simulink model "TestMultirotorSimPx4v1_8"  (R2018b)
settings: Solver=VariableStepAuto  StartTime=0.0  StopTime=Simulation.T_END  MaxStep=Simulation.TS_MAX  RelTol=1e-3  EnableMultiTasking=on
PreLoadFcn:
  | % InitializeParameters;
undefined symbols (not defined in the file): Aero, armed, ctrl_state, Initial, Motor, Simulation, Uav, v_att_sp, v_control_mode
libraries: QuaternionLibrary x13, simulink_extras x9, Px4Library x3, dspsigattribs x1, dspstat3 x1, simulink x1
(part 2 of 9)

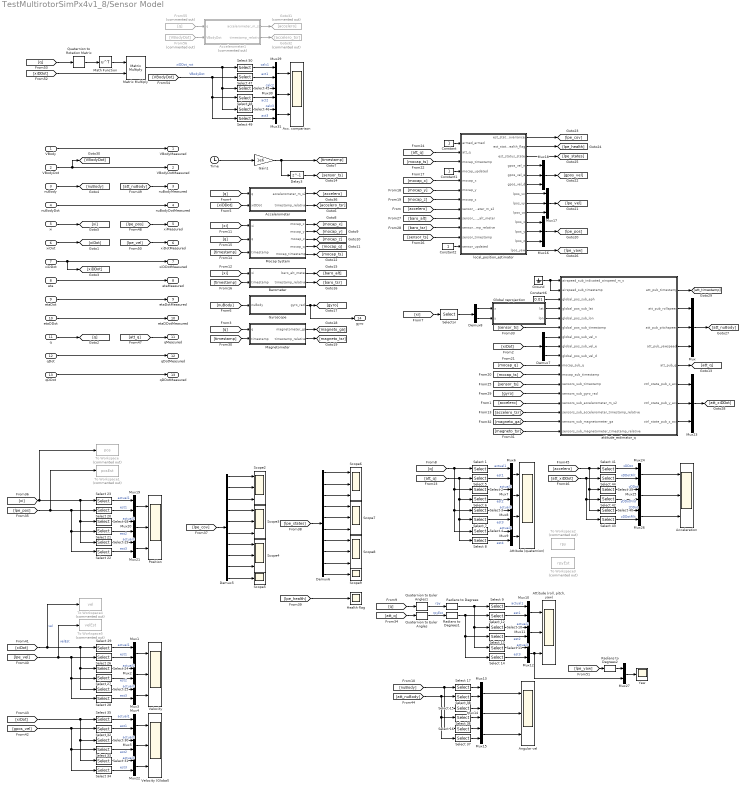
== system TestMultirotorSimPx4v1_8/Sensor Model ==
  VBody : Inport  Unit=m/s  PortDimensions=3
  VBodyDot : Inport  Port=2  Unit=m/s^2  PortDimensions=3
  nuBody : Inport  Port=3  Unit=rad/s  PortDimensions=3
  nuBodyDot : Inport  Port=4  Unit=rad/s^2  PortDimensions=3
  xi : Inport  Port=5  Unit=m  PortDimensions=3
  xiDot : Inport  Port=6  Unit=m/s  PortDimensions=3
  xiDDot : Inport  Port=7  Unit=m/s^2  PortDimensions=3
  eta : Inport  Port=8  Unit=rad  PortDimensions=3
  etaDot : Inport  Port=9  Unit=rad/s  PortDimensions=3
  etaDDot : Inport  Port=10  Unit=rad/s^2  PortDimensions=3
  q : Inport  Port=11  PortDimensions=4
  qDot : Inport  Port=12  PortDimensions=4
  qDDot : Inport  Port=13  PortDimensions=4
  Acc. comparison : Scope  NumInputPorts=3
  Acceleration : Scope  NumInputPorts=3
  Accelerometer : Subsystem
  Accelerometer1 : Subsystem  Commented=on
  Angular vel : Scope  NumInputPorts=3
  Attitude (quaternion) : Scope  NumInputPorts=4
  "Attitude (roll, pitch, yaw)" : Scope  NumInputPorts=3
  Barometer : Subsystem
  Constant : Constant
  Constant1 : Constant
  Constant2 : Constant
  Constant6 : Constant  Value=0.01
  Delay3 : Delay  DelayLength=1  SampleTime=1/400
  Demux5 : Demux  Outputs=10
  Demux6 : Demux  Outputs=10
  Demux7 : Demux  Outputs=3
  Demux8 : Demux  Outputs=2
  From55 : From  Commented=on  GotoTag=q
  From56 : From  Commented=on  GotoTag=VBodyDot
  Gain1 : Gain  Gain=1e6
  Global reprojection : Subsystem  AncestorBlock=Px4Library/Global reprojection  mask{LAT0=-36.865577, LON0=174.772065}
      mask prompts: LAT0 "Latitude at [x,y] = [0,0]"; LON0 "Longitude at [x,y] = [0,0]"
      mask Display:
      | disp('REPROJECT')
      | port_label('input', 1, sprintf('x'))
      | port_label('input', 2, sprintf('y'))
      | port_label('output', 1, sprintf('lat'))
      | port_label('output', 2, sprintf('lon'))
  Goto31 : Goto  Commented=on  GotoTag=accelero
  Goto32 : Goto  Commented=on  GotoTag=accelero_tsr
  Ground : Ground
  Gyroscope : Subsystem
  Health flag : Scope
  Magnetometer : Subsystem
  Math Function : Math  Operator=transpose  SaturateOnIntegerOverflow=on
  Matrix Multiply : Product  Multiplication=Matrix(*)
  Mocap System : Subsystem
  Mux{,16..18,23} (5 alike) : Mux  Inputs=3
  Mux{1..15,19..22,24..27,29..31} (26 alike) : Mux  Inputs=2
  Position : Scope  NumInputPorts=3
  Quaternion to Euler Angles : QuaternionLibrary/Quaternion to Euler Angles
  Quaternion to Euler Angles1 : QuaternionLibrary/Quaternion to Euler Angles
  Quaternion to Rotation Matrix : QuaternionLibrary/Quaternion to Rotation Matrix
  Radians to Degrees : simulink_extras/Transformations/Radians to Degrees
  Radians to Degrees1 : simulink_extras/Transformations/Radians to Degrees
  Radians to Degrees2 : simulink_extras/Transformations/Radians to Degrees
  Scope{2..4,6..8} (6 alike) : Scope  NumInputPorts=3
  Scope5 : Scope
  Scope9 : Scope
  Select 1 : Selector  InputPortWidth=4  IndexOptions=Index vector (dialog)  Indices=1  OutputSizes=1
  Select {10,13,15,18,21,24,27,30,33,36,39,42,45,48} (14 alike) : Selector  InputPortWidth=3  IndexOptions=Index vector (dialog)  Indices=2  OutputSizes=1
  Select {11,14,16,19,22,25,28,31,34,37,40,43,46,49} (14 alike) : Selector  InputPortWidth=3  IndexOptions=Index vector (dialog)  Indices=3  OutputSizes=1
  Select {9,12,17,20,23,26,29,32,35,38,41,44,47,50} (14 alike) : Selector  InputPortWidth=3  IndexOptions=Index vector (dialog)  Indices=1  OutputSizes=1
  Select 2 : Selector  InputPortWidth=4  IndexOptions=Index vector (dialog)  Indices=2  OutputSizes=1
  Select 3 : Selector  InputPortWidth=4  IndexOptions=Index vector (dialog)  Indices=3  OutputSizes=1
  Select 4 : Selector  InputPortWidth=4  IndexOptions=Index vector (dialog)  Indices=4  OutputSizes=1
  Select 5 : Selector  InputPortWidth=4  IndexOptions=Index vector (dialog)  Indices=1  OutputSizes=1
  Select 6 : Selector  InputPortWidth=4  IndexOptions=Index vector (dialog)  Indices=2  OutputSizes=1
  Select 7 : Selector  InputPortWidth=4  IndexOptions=Index vector (dialog)  Indices=3  OutputSizes=1
  Select 8 : Selector  InputPortWidth=4  IndexOptions=Index vector (dialog)  Indices=4  OutputSizes=1
  Selector : Selector  InputPortWidth=3  IndexOptions=Index vector (dialog)  Indices=[1 2]  OutputSizes=1
  Time : Clock
  To Workspace : ToWorkspace  Commented=on  VariableName=pos  SaveFormat=Structure With Time  SampleTime=-1
  To Workspace1 : ToWorkspace  Commented=on  VariableName=posEst  SaveFormat=Structure With Time  SampleTime=-1
  To Workspace2 : ToWorkspace  Commented=on  VariableName=rpy  SaveFormat=Structure With Time  SampleTime=-1
  To Workspace3 : ToWorkspace  Commented=on  VariableName=rpyEst  SaveFormat=Structure With Time  SampleTime=-1
  To Workspace4 : ToWorkspace  Commented=on  VariableName=vel  SaveFormat=Structure With Time  SampleTime=-1
  To Workspace5 : ToWorkspace  Commented=on  VariableName=velEst  SaveFormat=Structure With Time  SampleTime=-1
  Velocity : Scope  NumInputPorts=3
  Velocity (Global) : Scope  NumInputPorts=3
  Yaw : Scope
  attitude_estimator_q : Subsystem  AncestorBlock=Px4Library/attitude_estimator_q  mask(PX4 LPE (local position estimator): local_position_estimator){Q_SAMPLING_PERIOD=1/250, INIT_Q=[1  0  0  0], ATT_W_ACC=0.2, ATT_W_MAG=0.1, ATT_W_EXT_HDG=0.1, ATT_W_GYRO_BIAS=0.1, ATT_MAG_DECL=0.0, ATT_MAG_DECL_A=1, ATT_EXT_HDG_M=2, ATT_ACC_COMP=1, ATT_BIAS_MAX=0.05, FW_ARSP_MODE=0}
      mask prompts: Q_SAMPLING_PERIOD "Sampling period (s)"; INIT_Q "INIT_Q - Initial UAV orientation - set to 0 to let controller decide (bugged) (-)"; ATT_W_ACC "ATT_W_ACC - Complimentary filter accelerometer weight (-)"; ATT_W_MAG "ATT_W_MAG - Complimentary filter magnetometer weight (-)"; ATT_W_EXT_HDG "ATT_W_EXT_HDG - Complimentary filter external heading weight (-)"; ATT_W_GYRO_BIAS "ATT_W_GYRO_BIAS - Complimentary filter gyroscope bias weight (-)"; ATT_MAG_DECL "ATT_MAG_DECL - Magnetic declination. Not used when GPS available (deg)"; ATT_MAG_DECL_A "ATT_MAG_DECL_A - Automatic GPS based declination compensation (-)"; ATT_EXT_HDG_M "ATT_EXT_HDG_M - External heading usage mode (from Motion capture/Vision) (-), 0 None 1 Vision 2 Motion Capture"; ATT_ACC_COMP "ATT_ACC_COMP - Acceleration compensation based on GPS velocity. (-)"; ATT_BIAS_MAX "ATT_BIAS_MAX - Gyro bias limit (rad/s)"; FW_ARSP_MODE "FW_ARSP_MODE - Method used to publish the airspeed (-), 0 Measured airspeed 1 Vehicle ground speed 2 Airspeed invalid"
      mask TypeOptions ATT_EXT_HDG_M: 0 | 1 | 2
      mask TypeOptions FW_ARSP_MODE: 0 | 1 | 2
  local_position_estimator : Subsystem  AncestorBlock=Px4Library/local_position_estimator  mask(PX4 LPE (local position estimator): local_position_estimator){LPE_SAMPLING_PERIOD=0.01, LPE_ACC_XY=0.012, LPE_ACC_Z=0.02, LPE_BAR_Z=3, LPE_EPH_MAX=3, LPE_EPV_MAX=5, LPE_FAKE_ORIGIN=0, LPE_FGYRO_HP=0.001, LPE_FLW_OFF_Z=0, LPE_FLW_QMIN=150, LPE_FLW_R=7, LPE_FLW_RR=7, LPE_FLW_SCALE=1.3, LPE_GPS_DELAY=0.29, LPE_GPS_VXY=0.25, LPE_GPS_VZ=0.25, LPE_GPS_XY=1, LPE_GPS_Z=3, LPE_LAND_VXY=0.05, LPE_LAND_Z=0.03, LPE_LAT=47.3977, LPE_LDR_OFF_Z=0, LPE_LDR_Z=0.03, LPE_LON=8.5456, LPE_PN_B=0.001, LPE_PN_P=0.1, LPE_PN_T=0.001, LPE_PN_V=0.1, LPE_SNR_OFF_Z=0, LPE_SNR_Z=0.05, LPE_T_MAX_GRADE=1, LPE_VIC_P=0.001, LPE_VIS_DELAY=0.1, LPE_VIS_XY=0.1, LPE_VIS_Z=0.5, LPE_VXY_PUB=0.3, LPE_X_LP=5, LPE_Z_PUB=1, LPE_FUSION=193, Barometer=on, GPS=off, LIDAR=off, Flow=off, Sonar=off, Vision=off, Mocap=on, Land=on}
      mask prompts: LPE_SAMPLING_PERIOD "Sampling period (s)"; LPE_ACC_XY "LPE_ACC_XY - Accelerometer xy noise density (m/s^2/sqrt(Hz))"; LPE_ACC_Z "LPE_ACC_Z - Accelerometer z noise density (m/s^2/sqrt(Hz))"; LPE_BAR_Z "LPE_BAR_Z - Barometric presssure altitude z standard deviation. (m)"; LPE_EPH_MAX "LPE_EPH_MAX - Max EPH allowed for GPS initialization (m)"; LPE_EPV_MAX "LPE_EPV_MAX - Max EPV allowed for GPS initialization (m)"; LPE_FAKE_ORIGIN "LPE_FAKE_ORIGIN - Enable publishing of a fake global position (e.g for AUTO missions using Optical Flow) (-)"; LPE_FGYRO_HP "LPE_FGYRO_HP - Flow gyro high pass filter cut off frequency (Hz)"; LPE_FLW_OFF_Z "LPE_FLW_OFF_Z - Optical flow z offset from center (m)"; LPE_FLW_QMIN "LPE_FLW_QMIN - Optical flow minimum quality threshold (-)"; LPE_FLW_R "LPE_FLW_R - Optical flow rotation (roll/pitch) noise gain (m/s / (rad))"; LPE_FLW_RR "LPE_FLW_RR - Optical flow angular velocity noise gain (m/s / (rad/s))"; LPE_FLW_SCALE "LPE_FLW_SCALE - Optical flow scale (m)"; LPE_GPS_DELAY "LPE_GPS_DELAY - GPS delay compensaton (sec)"; LPE_GPS_VXY "LPE_GPS_VXY - GPS xy velocity standard deviation. (m/s)"; LPE_GPS_VZ "LPE_GPS_VZ - GPS z velocity standard deviation. (m/s)"; LPE_GPS_XY "LPE_GPS_XY - Minimum GPS xy standard deviation, uses reported EPH if greater. (m)"; LPE_GPS_Z "LPE_GPS_Z - Minimum GPS z standard deviation, uses reported EPV if greater. (m)"; LPE_LAND_VXY "LPE_LAND_VXY - Land detector xy velocity standard deviation (m/s)"; LPE_LAND_Z "LPE_LAND_Z - Land detector z standard deviation (m)"; LPE_LAT "LPE_LAT - Local origin latitude for nav w/o GPS (deg)"; LPE_LDR_OFF_Z "LPE_LDR_OFF_Z - Lidar z offset from center of vehicle +down (m)"; LPE_LDR_Z "LPE_LDR_Z - Lidar z standard deviation. (m)"; LPE_LON "LPE_LON - Local origin longitude for nav w/o GPS (deg)"; LPE_PN_B "LPE_PN_B - Accel bias propagation noise density ((m/s^2)/s/sqrt(Hz))"; LPE_PN_P "LPE_PN_P - Position propagation noise density (m/s/sqrt(Hz))"; LPE_PN_T "LPE_PN_T - Terrain random walk noise density, hilly/outdoor (0.1), flat/Indoor (0.001) ((m/s)/(sqrt(hz)))"; LPE_PN_V "LPE_PN_V - Velocity propagation noise density ((m/s)/s/sqrt(Hz))"; LPE_SNR_OFF_Z "LPE_SNR_OFF_Z - Sonar z offset from center of vehicle +down (m)"; LPE_SNR_Z "LPE_SNR_Z - Sonar z standard deviation. (m)"; LPE_T_MAX_GRADE "LPE_T_MAX_GRADE - Terrain maximum percent grade, hilly/outdoor (100 = 45 deg), flat/Indoor (0 = 0 deg) (%)"; LPE_VIC_P "LPE_VIC_P - Vicon position standard deviation. (m)"; LPE_VIS_DELAY "LPE_VIS_DELAY - Vision delay compensaton. (sec)"; LPE_VIS_XY "LPE_VIS_XY - Vision xy standard deviation. (m)"; LPE_VIS_Z "LPE_VIS_Z - Vision z standard deviation. (m)"; LPE_VXY_PUB "LPE_VXY_PUB - Required velocity xy standard deviation to publish position (m/s)"; LPE_X_LP "LPE_X_LP - Cut frequency for state publication (Hz)"; LPE_Z_PUB "LPE_Z_PUB - Required z standard deviation to publish altitude/ terrain (m)"; LPE_FUSION "LPE_FUSION - Integer bitmask controlling data fusion (-)"; Barometer "Use Barometer"; GPS "Use GPS"; LIDAR "Use LIDAR"; Flow "Use Flow"; Sonar "Use Sonar"; Vision "Use Vision"; Mocap "Use Mocap"; Land "Use Land"
      mask Callback Barometer:
      | status = get_param( gcb, 'Barometer' );
      | if strcmp( status, 'on' )
      | 	lpe = bitor( uint8(str2num(get_param( gcb, 'LPE_FUSION' ))), uint8(2^0) );
      | 	set_param( gcb, 'LPE_FUSION', num2str(lpe) );
      | else
      | 	lpe = bitand( uint8(str2num(get_param( gcb, 'LPE_FUSION' ))), bitcmp(uint8(2^0), 'uint8' ));
      | 	set_param( gcb, 'LPE_FUSION', num2str(lpe) );
      | end
      mask Callback GPS:
      | status = get_param( gcb, 'GPS' );
      | if strcmp( status, 'on' )
      | 	lpe = bitor( uint8(str2num(get_param( gcb, 'LPE_FUSION' ))), uint8(2^1) );
      | 	set_param( gcb, 'LPE_FUSION', num2str(lpe) );
      | else
      | 	lpe = bitand( uint8(str2num(get_param( gcb, 'LPE_FUSION' ))), bitcmp(uint8(2^1), 'uint8' ));
      | 	set_param( gcb, 'LPE_FUSION', num2str(lpe) );
      | end
      mask Callback LIDAR:
      | status = get_param( gcb, 'LIDAR' );
      | if strcmp( status, 'on' )
      | 	lpe = bitor( uint8(str2num(get_param( gcb, 'LPE_FUSION' ))), uint8(2^2) );
      | 	set_param( gcb, 'LPE_FUSION', num2str(lpe) );
      | else
      | 	lpe = bitand( uint8(str2num(get_param( gcb, 'LPE_FUSION' ))), bitcmp(uint8(2^2), 'uint8' ));
      | 	set_param( gcb, 'LPE_FUSION', num2str(lpe) );
      | end
      mask Callback Flow:
      | status = get_param( gcb, 'Flow' );
      | if strcmp( status, 'on' )
      | 	lpe = bitor( uint8(str2num(get_param( gcb, 'LPE_FUSION' ))), uint8(2^3) );
      | 	set_param( gcb, 'LPE_FUSION', num2str(lpe) );
      | else
      | 	lpe = bitand( uint8(str2num(get_param( gcb, 'LPE_FUSION' ))), bitcmp(uint8(2^3), 'uint8' ));
      | 	set_param( gcb, 'LPE_FUSION', num2str(lpe) );
      | end
      mask Callback Sonar:
      | status = get_param( gcb, 'Sonar' );
      | if strcmp( status, 'on' )
      | 	lpe = bitor( uint8(str2num(get_param( gcb, 'LPE_FUSION' ))), uint8(2^4) );
      | 	set_param( gcb, 'LPE_FUSION', num2str(lpe) );
      | else
      | 	lpe = bitand( uint8(str2num(get_param( gcb, 'LPE_FUSION' ))), bitcmp(uint8(2^4), 'uint8' ));
      | 	set_param( gcb, 'LPE_FUSION', num2str(lpe) );
      | end
      mask Callback Vision:
      | status = get_param( gcb, 'Vision' );
      | if strcmp( status, 'on' )
      | 	lpe = bitor( uint8(str2num(get_param( gcb, 'LPE_FUSION' ))), uint8(2^5) );
      | 	set_param( gcb, 'LPE_FUSION', num2str(lpe) );
      | else
      | 	lpe = bitand( uint8(str2num(get_param( gcb, 'LPE_FUSION' ))), bitcmp(uint8(2^5), 'uint8' ));
      | 	set_param( gcb, 'LPE_FUSION', num2str(lpe) );
      | end
      mask Callback Mocap:
      | status = get_param( gcb, 'Mocap' );
      | if strcmp( status, 'on' )
      | 	lpe = bitor( uint8(str2num(get_param( gcb, 'LPE_FUSION' ))), uint8(2^6) );
      | 	set_param( gcb, 'LPE_FUSION', num2str(lpe) );
      | else
      | 	lpe = bitand( uint8(str2num(get_param( gcb, 'LPE_FUSION' ))), bitcmp(uint8(2^6), 'uint8' ));
      | 	set_param( gcb, 'LPE_FUSION', num2str(lpe) );
      | end
      mask Callback Land:
      | status = get_param( gcb, 'Land' );
      | if strcmp( status, 'on' )
      | 	lpe = bitor( uint8(str2num(get_param( gcb, 'LPE_FUSION' ))), uint8(2^7) );
      | 	set_param( gcb, 'LPE_FUSION', num2str(lpe) );
      | else
      | 	lpe = bitand( uint8(str2num(get_param( gcb, 'LPE_FUSION' ))), bitcmp(uint8(2^7), 'uint8' ));
      | 	set_param( gcb, 'LPE_FUSION', num2str(lpe) );
      | end
  VBodyMeasured : Outport  Unit=m/s
  VBodyDotMeasured : Outport  Port=2  Unit=m/s^2
  nuBodyMeasured : Outport  Port=3  Unit=rad/s
  nuBodyDotMeasured : Outport  Port=4  Unit=rad/s^2
  xiMeasured : Outport  Port=5  Unit=m
  xiDotMeasured : Outport  Port=6  Unit=m/s
  xiDDotMeasured : Outport  Port=7  Unit=m/s^2
  etaMeasured : Outport  Port=8  Unit=rad
  etaDotMeasured : Outport  Port=9  Unit=rad/s
  etaDDotMeasured : Outport  Port=10  Unit=rad/s^2
  qMeasured : Outport  Port=11
  qDotMeasured : Outport  Port=12
  qDDotMeasured : Outport  Port=13
  gyro : Outport  Port=14
  wires:
  xiDot/1 -> [xiDot]
  xi/1 -> [xi]
  nuBodyDot/1 -> nuBodyDotMeasured/1
  nuBody/1 -> [nuBody]
  VBodyDot/1 -> [VBodyDot], VBodyDotMeasured/1
  VBody/1 -> VBodyMeasured/1
  eta/1 -> etaMeasured/1
  etaDot/1 -> etaDotMeasured/1
  etaDDot/1 -> etaDDotMeasured/1
  q/1 -> [q]
  qDot/1 -> qDotMeasured/1
  qDDot/1 -> qDDotMeasured/1
  [att_q] -> local_position_estimator/2(att_q)
  [mocap_x] -> local_position_estimator/5(mocap_x)
  [mocap_z] -> local_position_estimator/7(mocap_z)
  local_position_estimator/10(lpos_x) -> Mux16/1
  local_position_estimator/11(lpos_y) -> Mux16/2
  local_position_estimator/12(lpos_z) -> Mux16/3
  Demux5/2 -> Scope2/2
  Demux5/1 -> Scope2/1
  Demux5/3 -> Scope2/3
  Demux5/4 -> Scope3/1
  Demux5/5 -> Scope3/2
  Demux5/6 -> Scope3/3
  Demux5/7 -> Scope4/1
  Demux5/8 -> Scope4/2
  Demux5/9 -> Scope4/3
  Demux5/10 -> Scope5/1
  [lpe_states] -> Demux6/1
  Demux6/2 -> Scope6/2
  Demux6/1 -> Scope6/1
  Demux6/3 -> Scope6/3
  Demux6/4 -> Scope7/1
  Demux6/5 -> Scope7/2
  Demux6/6 -> Scope7/3
  Demux6/7 -> Scope8/1
  Demux6/8 -> Scope8/2
  Demux6/9 -> Scope8/3
  Demux6/10 -> Scope9/1
  Constant1/1 -> local_position_estimator/4(mocap_updated)
  [lpe_health] -> Health flag/1
  Constant/1 -> local_position_estimator/1(armed_armed)
  [mocap_ts] -> local_position_estimator/3(mocap_timestamp)
  [xiDot] -> Demux7/1
  Time/1 -> Gain1/1
  [accelero_tsr] -> attitude_estimator_q/15(sensors_sub_accelerometer_timestamp_relative)
  Global reprojection/1(lat) -> attitude_estimator_q/4(global_pos_sub_lat)
  Global reprojection/2(lon) -> attitude_estimator_q/5(global_pos_sub_lon)
  [xi] -> Selector/1
  Selector/1 -> Demux8/1
  Demux8/1 -> Global reprojection/1(x)
  Demux8/2 -> Global reprojection/2(y)
  [att_q] -> Select 8/1, Select 7/1, Select 6/1, Select 5/1
  [q] -> Select 2/1, Select 3/1, Select 4/1, Select 1/1
  Mux6/1 -> Attitude (quaternion)/1
  Mux7/1 -> Attitude (quaternion)/2
  Mux8/1 -> Attitude (quaternion)/3
  Mux9/1 -> Attitude (quaternion)/4
  Select 4/1 -> Mux9/1  "actual4"
  Select 8/1 -> Mux9/2  "est4"
  Select 3/1 -> Mux8/1  "actual3"
  Select 7/1 -> Mux8/2  "est3"
  Select 6/1 -> Mux7/2  "est2"
  Select 2/1 -> Mux7/1  "actual2"
  Select 5/1 -> Mux6/2  "est1"
  Select 1/1 -> Mux6/1  "actual1"
  Constant6/1 -> attitude_estimator_q/3(global_pos_sub_eph)
  [q] -> Magnetometer/1(q)
  Mux10/1 -> "Attitude (roll, pitch, yaw)"/1
  Mux11/1 -> "Attitude (roll, pitch, yaw)"/2
  Mux12/1 -> Mux27/2, "Attitude (roll, pitch, yaw)"/3
  Select 11/1 -> Mux12/1  "actual3"
  Select 14/1 -> Mux12/2  "est3"
  Select 13/1 -> Mux11/2  "est2"
  Select 10/1 -> Mux11/1  "actual2"
  Select 12/1 -> Mux10/2  "est1"
  Select 9/1 -> Mux10/1  "actual1"
  [q] -> Quaternion to Euler Angles1/1
  Quaternion to Euler Angles1/1 -> Radians to Degrees/1  "rpy"
  Quaternion to Euler Angles/1 -> Radians to Degrees1/1  "rpyEst"
  Mux13/1 -> Angular vel/1
  Mux14/1 -> Angular vel/2
  Mux15/1 -> Angular vel/3
  Select 17/1 -> Mux13/1
  Select 15/1 -> Mux14/1
  Select 16/1 -> Mux15/1
  [nuBody] -> Select 17/1, Select 16/1, Select 15/1
  Demux7/2 -> attitude_estimator_q/8(global_pos_sub_vel_e)
  [accelero] -> attitude_estimator_q/14(sensors_sub_accelerometer_m_s2)
  [sensor_ts] -> attitude_estimator_q/12(sensors_sub_timestamp)
  [magneto_ga] -> attitude_estimator_q/16(sensors_sub_magnetometer_ga)
  [nuBody] -> Gyroscope/1(nuBody)
  [gyro] -> attitude_estimator_q/13(sensors_sub_gyro_rad)
  [q] -> Accelerometer/1(q)
  [xiDDot] -> Accelerometer/2(xiDDot)
  Accelerometer/1(accelerometer_m_s2) -> [accelero]
  Accelerometer/2(timestamp_relative) -> [accelero_tsr]
  [mocap_q] -> attitude_estimator_q/10(mocap_sub_q)
  [mocap_ts] -> attitude_estimator_q/11(mocap_sub_timestamp)
  Gain1/1 -> Delay3/1, [timestamp]
  [timestamp] -> Mocap System/3(timestamp)
  [q] -> Mocap System/2(q)
  [xi] -> Mocap System/1(xi)
  Constant2/1 -> local_position_estimator/12(sensor_updated)
  [baro_alt] -> local_position_estimator/9(sensor_baro_alt_meter)
  [baro_tsr] -> local_position_estimator/10(sensor_baro_timestamp_relative)
  Mocap System/1(mocap_x) -> [mocap_x]
  Mocap System/2(mocap_y) -> [mocap_y]
  Mocap System/3(mocap_z) -> [mocap_z]
  [mocap_y] -> local_position_estimator/6(mocap_y)
  Mocap System/4(mocap_q) -> [mocap_q]
  Mocap System/5(mocap_timestamp) -> [mocap_ts]
  attitude_estimator_q/5(att_pub_q) -> [att_q]
  Delay3/1 -> [sensor_ts]
  [sensor_ts] -> local_position_estimator/11(sensor_timestamp)
  [xi] -> Barometer/1(xi)
  [timestamp] -> Barometer/2(timestamp)
  Barometer/1(baro_alt_meter) -> [baro_alt]
  Barometer/2(timestamp_relative) -> [baro_tsr]
  Gyroscope/1(gyro_rad) -> gyro/1, [gyro]
  [timestamp] -> Magnetometer/2(timestamp)
  Magnetometer/2(timestamp_relative) -> [magneto_tsr]
  Magnetometer/1(magnetometer_ga) -> [magneto_ga]
  [magneto_tsr] -> attitude_estimator_q/17(sensors_sub_magnetometer_timestamp_relative)
  Demux7/1 -> attitude_estimator_q/7(global_pos_sub_vel_n)
  Demux7/3 -> attitude_estimator_q/9(global_pos_sub_vel_d)
  [sensor_ts] -> attitude_estimator_q/6(global_pos_sub_timestamp)
  Mux16/1 -> [lpe_pos]
  local_position_estimator/7(lpos_vx) -> Mux17/1
  local_position_estimator/8(lpos_vy) -> Mux17/2
  local_position_estimator/9(lpos_vz) -> Mux17/3
  Mux17/1 -> [lpe_vel]
  local_position_estimator/4(gpos_vel_n) -> Mux18/1
  local_position_estimator/5(gpos_vel_e) -> Mux18/2
  local_position_estimator/6(gpos_vel_d) -> Mux18/3
  Mux18/1 -> [gpos_vel]
  local_position_estimator/1(est_status_covariances) -> [lpe_cov]
  local_position_estimator/2(est_status_health_flags) -> [lpe_health]
  local_position_estimator/3(est_status_states) -> [lpe_states]
  [att_q] -> Quaternion to Euler Angles/1
  Mux19/1 -> Position/1
  Mux20/1 -> Position/2
  Mux21/1 -> Position/3
  Select 19/1 -> Mux21/1  "actual3"
  Select 22/1 -> Mux21/2  "est3"
  Select 21/1 -> Mux20/2  "est2"
  Select 18/1 -> Mux20/1  "actual2"
  Select 20/1 -> Mux19/2  "est1"
  Select 23/1 -> Mux19/1  "actual1"
  [lpe_pos] -> To Workspace1/1, Select 20/1, Select 21/1, Select 22/1
  [lpe_cov] -> Demux5/1
  [xi] -> Select 23/1, Select 18/1, Select 19/1, To Workspace/1
  Mux1/1 -> Velocity/1
  Mux2/1 -> Velocity/2
  Mux3/1 -> Velocity/3
  Select 25/1 -> Mux3/1  "actual3"
  Select 28/1 -> Mux3/2  "est3"
  Select 27/1 -> Mux2/2  "est2"
  Select 24/1 -> Mux2/1  "actual2"
  Select 26/1 -> Mux1/2  "est1"
  Select 29/1 -> Mux1/1  "actual1"
  [lpe_vel] -> To Workspace5/1, Select 28/1, Select 27/1, Select 26/1  "velEst"
  [xiDot] -> To Workspace4/1, Select 25/1, Select 24/1, Select 29/1  "vel"
  Mux4/1 -> Velocity (Global)/1
  Mux5/1 -> Velocity (Global)/2
  Mux22/1 -> Velocity (Global)/3
  Select 31/1 -> Mux22/1  "actual3"
  Select 34/1 -> Mux22/2  "est3"
  Select 33/1 -> Mux5/2  "est2"
  Select 30/1 -> Mux5/1  "actual2"
  Select 32/1 -> Mux4/2  "est1"
  Select 35/1 -> Mux4/1  "actual1"
  [gpos_vel] -> Select 32/1, Select 33/1, Select 34/1
  [xiDot] -> Select 35/1, Select 30/1, Select 31/1
  [accelero] -> local_position_estimator/8(sensor_accelerometer_m_s2)
  local_position_estimator/13(lpos_yaw) -> [lpe_yaw]
  Mux/1 -> [att_nuBody]
  attitude_estimator_q/3(att_pub_pitchspeed) -> Mux/2
  attitude_estimator_q/2(att_pub_rollspeed) -> Mux/1
  attitude_estimator_q/4(att_pub_yawspeed) -> Mux/3
  Select 38/1 -> Mux13/2
  Select 37/1 -> Mux15/2
  [att_nuBody] -> Select 38/1, Select 36/1, Select 37/1
  Select 36/1 -> Mux14/2
  Mux23/1 -> [att_xiDDot]
  attitude_estimator_q/7(ctrl_state_pub_y_acc) -> Mux23/2
  attitude_estimator_q/6(ctrl_state_pub_x_acc) -> Mux23/1
  attitude_estimator_q/8(ctrl_state_pub_z_acc) -> Mux23/3
  Mux24/1 -> Acceleration/1
  Mux25/1 -> Acceleration/2
  Mux26/1 -> Acceleration/3
  Select 41/1 -> Mux24/1  "xDDot"
  Select 39/1 -> Mux25/1  "yDDot"
  Select 40/1 -> Mux26/1  "zDDot"
  [accelero] -> Select 39/1, Select 40/1, Select 41/1
  Select 44/1 -> Mux24/2  "xDDotFilt"
  Select 43/1 -> Mux26/2  "zDDotFilt"
  [att_xiDDot] -> Select 43/1, Select 42/1, Select 44/1
  Select 42/1 -> Mux25/2  "yDDotFild"
  attitude_estimator_q/1(att_pub_timestamp) -> [att_timestamp]
  [att_q] -> qMeasured/1
  [att_nuBody] -> nuBodyMeasured/1
  xiDDot/1 -> xiDDotMeasured/1, [xiDDot]
  [lpe_pos] -> xiMeasured/1
  [lpe_vel] -> xiDotMeasured/1
  Ground/1 -> attitude_estimator_q/2(airspeed_sub_timestamp), attitude_estimator_q/1(airspeed_sub_indicated_airspeed_m_s)
  [lpe_yaw] -> Radians to Degrees2/1
  Mux27/1 -> Yaw/1
  Quaternion to Rotation Matrix/1 -> Math Function/1
  Math Function/1 -> Matrix Multiply/1
  [q] -> Quaternion to Rotation Matrix/1
  [xiDDot] -> Matrix Multiply/2
  Matrix Multiply/1 -> Select 46/1, Select 45/1, Select 50/1  "xiDDot_rot"
  [VBodyDot] -> Select 49/1, Select 48/1, Select 47/1  "VBodyDot"
  Mux31/1 -> Acc. comparison/3
  Mux29/1 -> Acc. comparison/1
  Select 46/1 -> Mux31/1  "calc3"
  Select 45/1 -> Mux30/1  "calc2"
  Select 50/1 -> Mux29/1  "calc1"
  Mux30/1 -> Acc. comparison/2
  Select 48/1 -> Mux30/2  "act2"
  Select 49/1 -> Mux31/2  "act3"
  Select 47/1 -> Mux29/2  "act1"
  Accelerometer1/2(timestamp_relative) -> Goto32/1
  Accelerometer1/1(accelerometer_m_s2) -> Goto31/1
  From55/1 -> Accelerometer1/1(q)
  From56/1 -> Accelerometer1/2(VBodyDot)
  Radians to Degrees/1 -> Select 11/1, Select 10/1, Select 9/1
  Radians to Degrees1/1 -> Select 14/1, Select 13/1, Select 12/1
  Radians to Degrees2/1 -> Mux27/1

== system TestMultirotorSimPx4v1_8/Stick logging buffer ==
  stickIn : Inport
  stickOut : Outport
  wires:
  stickIn/1 -> stickOut/1

== system TestMultirotorSimPx4v1_8/att_mixerInput ==
  qPosCtrl : Inport
  qInput : Inport  Port=2
  Euler Angles to Quaternion : Subsystem  AncestorBlock=QuaternionLibrary/Euler Angles to Quaternion
      mask help: Convert vector of Euler angles to an orientation quaternion
      mask Help:
      | Convert vector of Euler angles
      | [roll, pitch, yaw]
      | to an orientation quaternion
      | [q1 q2 q3 q4]
      | where:
      | - q1 is the rotation in radians
      | - [q2 q3 q4] is the vector around which the rotation is performed)
      | 
      | Based on code from the PX4 firmware: https://github.com/PX4/Firmware
      mask Display: disp('E2Q')
  Mux : Mux  Inputs=3
  Quaternion to Euler Angles2 : Subsystem  AncestorBlock=QuaternionLibrary/Quaternion to Euler Angles
      mask help: Convert an orientation quaternion to a vector of Euler angles
      mask Help:
      | Convert an orientation quaternion
      | [q1 q2 q3 q4]
      | where:
      | - q1 is the rotation in radians
      | - [q2 q3 q4] is the vector around which the rotation is performed)
      | to a vector of Euler angles
      | [roll, pitch, yaw]
      | Based on code from the PX4 firmware: https://github.com/PX4/Firmware
      mask Display: disp('Q2E')
  Quaternion to Euler Angles3 : Subsystem  AncestorBlock=QuaternionLibrary/Quaternion to Euler Angles
      mask help: Convert an orientation quaternion to a vector of Euler angles
      mask Help:
      | Convert an orientation quaternion
      | [q1 q2 q3 q4]
      | where:
      | - q1 is the rotation in radians
      | - [q2 q3 q4] is the vector around which the rotation is performed)
      | to a vector of Euler angles
      | [roll, pitch, yaw]
      | Based on code from the PX4 firmware: https://github.com/PX4/Firmware
      mask Display: disp('Q2E')
  Selector25 : Selector  InputPortWidth=3  IndexOptions=Index vector (dialog)  Indices=1  OutputSizes=1
  Selector27 : Selector  InputPortWidth=3  IndexOptions=Index vector (dialog)  Indices=3  OutputSizes=1
  Selector28 : Selector  InputPortWidth=3  IndexOptions=Index vector (dialog)  Indices=2  OutputSizes=1
  qDes : Outport
  wires:
  qPosCtrl/1 -> Quaternion to Euler Angles2/1(quaternion)
  qInput/1 -> Quaternion to Euler Angles3/1(quaternion)
  Euler Angles to Quaternion/1(quaternion) -> qDes/1
  Mux/1 -> Euler Angles to Quaternion/1(euler)
  Quaternion to Euler Angles2/1(euler) -> Selector25/1
  Quaternion to Euler Angles3/1(euler) -> Selector27/1, Selector28/1
  Selector25/1 -> Mux/1
  Selector27/1 -> Mux/3
  Selector28/1 -> Mux/2

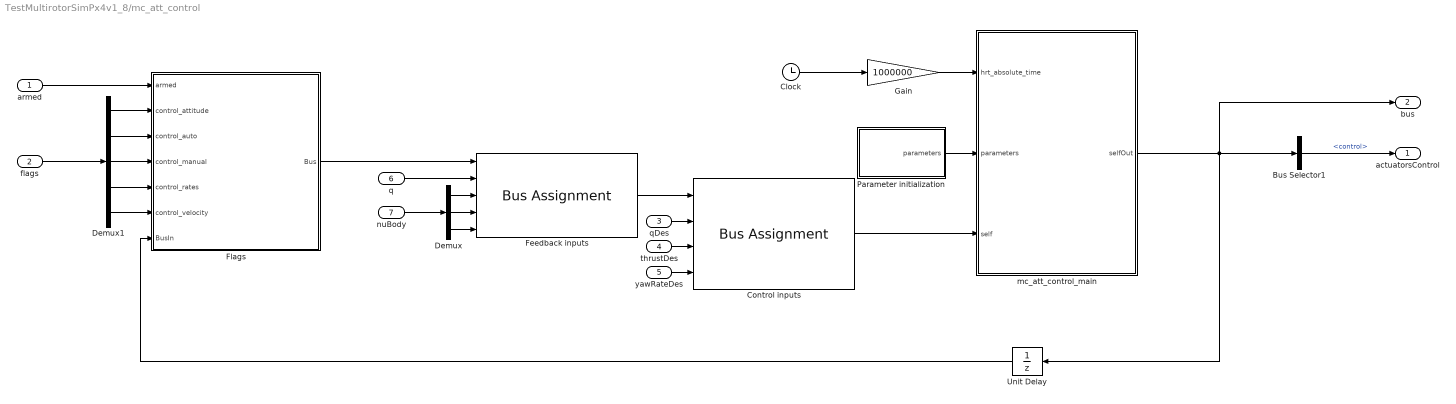
== system TestMultirotorSimPx4v1_8/mc_att_control ==
  armed : Inport  PortDimensions=1  SampleTime=MC_SAMPLING_PERIOD
  flags : Inport  Port=2  PortDimensions=5  SampleTime=MC_SAMPLING_PERIOD
  qDes : Inport  Port=3  PortDimensions=4  SampleTime=MC_SAMPLING_PERIOD
  thrustDes : Inport  Port=4  PortDimensions=1  SampleTime=MC_SAMPLING_PERIOD
  yawRateDes : Inport  Port=5  PortDimensions=1  SampleTime=MC_SAMPLING_PERIOD
  q : Inport  Port=6  PortDimensions=4  SampleTime=MC_SAMPLING_PERIOD
  nuBody : Inport  Port=7  PortDimensions=3  SampleTime=MC_SAMPLING_PERIOD
  Bus Selector1 : BusSelector  OutputSignals=actuators.control
  Clock : Clock
  Control inputs : BusAssignment  AssignedSignals=v_att_sp.q_d,v_att_sp.thrust,v_att_sp.yaw_sp_move_rate
  Demux : Demux  Outputs=3
  Demux1 : Demux  Outputs=5
  Feedback inputs : BusAssignment  AssignedSignals=ctrl_state.q,ctrl_state.roll_rate,ctrl_state.pitch_rate,ctrl_state.yaw_rate
  Flags : Subsystem
  Gain : Gain  Gain=1000000
  Parameter initialization : Subsystem
  Unit Delay : UnitDelay  SampleTime=MC_SAMPLING_PERIOD
  mc_att_control_main : MATLAB Function  TreatAsAtomicUnit=on  SystemSampleTime=MC_SAMPLING_PERIOD
  actuatorsControl : Outport  SampleTime=MC_SAMPLING_PERIOD
  bus : Outport  Port=2  SampleTime=MC_SAMPLING_PERIOD
  wires:
  flags/1 -> Demux1/1
  nuBody/1 -> Demux/1
  q/1 -> Feedback inputs/2
  armed/1 -> Flags/1(armed)
  Demux1/1 -> Flags/2(control_attitude)
  Demux1/2 -> Flags/3(control_auto)
  Demux1/3 -> Flags/4(control_manual)
  Demux1/4 -> Flags/5(control_rates)
  Demux1/5 -> Flags/6(control_velocity)
  yawRateDes/1 -> Control inputs/4
  thrustDes/1 -> Control inputs/3
  qDes/1 -> Control inputs/2
  Feedback inputs/1 -> Control inputs/1
  Gain/1 -> mc_att_control_main/1(hrt_absolute_time)
  Clock/1 -> Gain/1
  Demux/3 -> Feedback inputs/5
  Demux/2 -> Feedback inputs/4
  Demux/1 -> Feedback inputs/3
  Flags/1(Bus) -> Feedback inputs/1
  Control inputs/1 -> mc_att_control_main/3(self)
  Unit Delay/1 -> Flags/7(BusIn)
  Bus Selector1/1 -> actuatorsControl/1  "<control>"
  Parameter initialization/1(parameters) -> mc_att_control_main/2(parameters)
  mc_att_control_main/1(selfOut) -> Bus Selector1/1, Unit Delay/1, bus/1

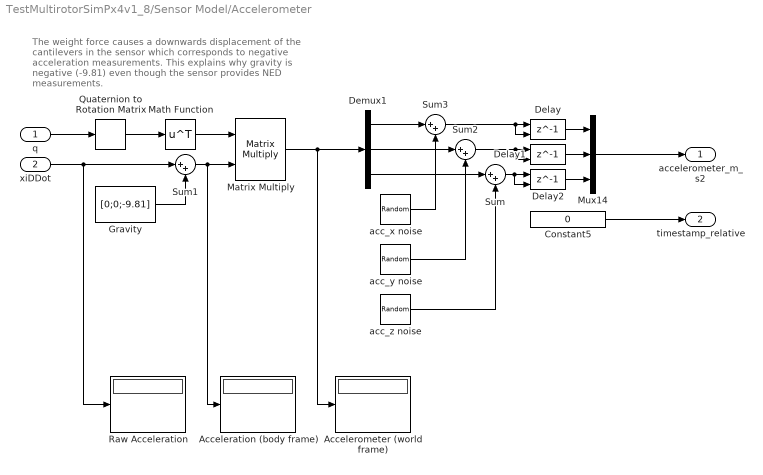
== system TestMultirotorSimPx4v1_8/Sensor Model/Accelerometer ==
  note: The weight force causes a downwards displacement of
      | the cantilevers in the sensor which corresponds to
      | negative acceleration measurements. This explains why
      | gravity is negative (-9.81) even though the sensor provides
      | NED measurements.
  q : Inport
  xiDDot : Inport  Port=2  Unit=m/s^2
  Acceleration (body frame) : Display
  Accelerometer (world frame) : Display
  Constant5 : Constant  Value=0
  Delay : Delay  DelayLength=1  InitialConditionSource=Input port  SampleTime=1/400
      settings: InputPortMap=u0,p4
  Delay1 : Delay  DelayLength=1  InitialConditionSource=Input port  SampleTime=1/400
      settings: InputPortMap=u0,p4
  Delay2 : Delay  DelayLength=1  InitialConditionSource=Input port  SampleTime=1/400
      settings: InputPortMap=u0,p4
  Demux1 : Demux  Outputs=3
  Gravity : Constant  Value=[0;0;-9.81]
  Math Function : Math  Operator=transpose  SaturateOnIntegerOverflow=on
  Matrix Multiply : Product  Multiplication=Matrix(*)
  Mux14 : Mux  Inputs=3
  Quaternion to Rotation Matrix : QuaternionLibrary/Quaternion to Rotation Matrix
  Raw Acceleration : Display
  Sum{,1..3} (4 alike) : Sum  Inputs=|++
  acc_x noise : RandomNumber  Variance=0.012^2  SampleTime=1/400
  acc_y noise : RandomNumber  Variance=0.012^2  SampleTime=1/400
  acc_z noise : RandomNumber  Variance=0.02^2  SampleTime=1/400
  accelerometer_m_s2 : Outport  Unit=m/s^2  SampleTime=1/400
  timestamp_relative : Outport  Port=2  Unit=µs  SampleTime=1/400
  wires:
  Quaternion to Rotation Matrix/1 -> Math Function/1
  Math Function/1 -> Matrix Multiply/1
  Matrix Multiply/1 -> Demux1/1, Accelerometer (world frame)/1
  Gravity/1 -> Sum1/2
  Sum1/1 -> Acceleration (body frame)/1, Matrix Multiply/2
  Mux14/1 -> accelerometer_m_s2/1
  q/1 -> Quaternion to Rotation Matrix/1
  Constant5/1 -> timestamp_relative/1
  Demux1/1 -> Sum3/1
  Demux1/2 -> Sum2/1
  Demux1/3 -> Sum/1
  Sum/1 -> Delay2/2, Delay2/1
  acc_z noise/1 -> Sum/2
  Sum2/1 -> Delay1/2, Delay1/1
  Sum3/1 -> Delay/2, Delay/1
  acc_y noise/1 -> Sum2/2
  acc_x noise/1 -> Sum3/2
  Delay/1 -> Mux14/1
  Delay1/1 -> Mux14/2
  Delay2/1 -> Mux14/3
  xiDDot/1 -> Sum1/1, Raw Acceleration/1

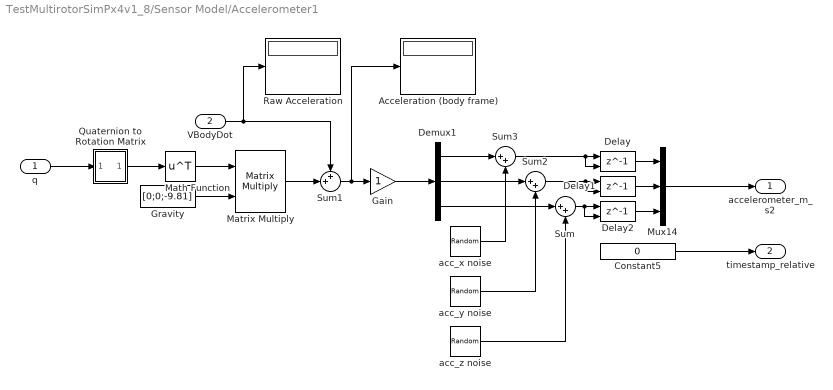
== system TestMultirotorSimPx4v1_8/Sensor Model/Accelerometer1 ==
  q : Inport
  VBodyDot : Inport  Port=2  Unit=m/s^2
  Acceleration (body frame) : Display
  Constant5 : Constant  Value=0
  Delay : Delay  DelayLength=1  InitialConditionSource=Input port  SampleTime=1/400
      settings: InputPortMap=u0,p4
  Delay1 : Delay  DelayLength=1  InitialConditionSource=Input port  SampleTime=1/400
      settings: InputPortMap=u0,p4
  Delay2 : Delay  DelayLength=1  InitialConditionSource=Input port  SampleTime=1/400
      settings: InputPortMap=u0,p4
  Demux1 : Demux  Outputs=3
  Gain : Gain
  Gravity : Constant  Value=[0;0;-9.81]
  Math Function : Math  Operator=transpose  SaturateOnIntegerOverflow=on
  Matrix Multiply : Product  Multiplication=Matrix(*)
  Mux14 : Mux  Inputs=3
  Quaternion to Rotation Matrix : Subsystem  AncestorBlock=QuaternionLibrary/Quaternion to Rotation Matrix
      mask help: Convert an orientation quaternion to an orthogonal transformation matrix
      mask Help:
      | Convert an orientation quaternion
      | [q1 q2 q3 q4]
      | where:
      | - q1 is the rotation in radians
      | - [q2 q3 q4] is the vector around which the rotation is performed)
      | to an orthogonal transformation matrix
      | Based on code from the PX4 firmware: https://github.com/PX4/Firmware
      mask Display: disp('Q2R')
  Raw Acceleration : Display
  Sum : Sum  Inputs=|++
  Sum1 : Sum  Inputs=++|
  Sum2 : Sum  Inputs=|++
  Sum3 : Sum  Inputs=|++
  acc_x noise : RandomNumber  Variance=0.012^2  SampleTime=1/400
  acc_y noise : RandomNumber  Variance=0.012^2  SampleTime=1/400
  acc_z noise : RandomNumber  Variance=0.02^2  SampleTime=1/400
  accelerometer_m_s2 : Outport  Unit=m/s^2  SampleTime=1/400
  timestamp_relative : Outport  Port=2  Unit=µs  SampleTime=1/400
  wires:
  Quaternion to Rotation Matrix/1(rotationMatrix) -> Math Function/1
  Math Function/1 -> Matrix Multiply/1
  Matrix Multiply/1 -> Sum1/2
  Gravity/1 -> Matrix Multiply/2
  Mux14/1 -> accelerometer_m_s2/1
  q/1 -> Quaternion to Rotation Matrix/1(quaternion)
  Constant5/1 -> timestamp_relative/1
  Demux1/1 -> Sum3/1
  Demux1/2 -> Sum2/1
  Demux1/3 -> Sum/1
  Sum/1 -> Delay2/2, Delay2/1
  acc_z noise/1 -> Sum/2
  Sum2/1 -> Delay1/2, Delay1/1
  Sum3/1 -> Delay/2, Delay/1
  acc_y noise/1 -> Sum2/2
  acc_x noise/1 -> Sum3/2
  Delay/1 -> Mux14/1
  Delay1/1 -> Mux14/2
  Delay2/1 -> Mux14/3
  Sum1/1 -> Acceleration (body frame)/1, Gain/1
  VBodyDot/1 -> Raw Acceleration/1, Sum1/1
  Gain/1 -> Demux1/1

== system TestMultirotorSimPx4v1_8/Sensor Model/Barometer ==
  xi : Inport  Unit=m
  timestamp : Inport  Port=2  Unit=µs
  Add : Sum  Inputs=+-
  Scope : Scope
  Select altitude : Selector  InputPortWidth=3  IndexOptions=Index vector (dialog)  Indices=3  OutputSizes=1
  Sum : Sum  Inputs=|++
  To 400 Hz : RateTransition  Deterministic=off  OutPortSampleTime=1/250
  To 400 Hz1 : RateTransition  OutPortSampleTime=1/400
  To 50 Hz : RateTransition  OutPortSampleTime=1/50
  To 50 Hz1 : RateTransition  OutPortSampleTime=1/50
  barro noise : RandomNumber  Variance=1/3^2  SampleTime=0.01
  baro_alt_meter : Outport  Unit=m  SampleTime=1/400
  timestamp_relative : Outport  Port=2  Unit=µs
  wires:
  barro noise/1 -> Sum/2
  Sum/1 -> To 50 Hz1/1
  xi/1 -> Select altitude/1
  Select altitude/1 -> Sum/1
  Add/1 -> timestamp_relative/1, Scope/1
  To 400 Hz1/1 -> Add/2
  To 50 Hz/1 -> To 400 Hz/1
  To 400 Hz/1 -> Add/1
  timestamp/1 -> To 50 Hz/1, To 400 Hz1/1
  To 50 Hz1/1 -> baro_alt_meter/1

== system TestMultirotorSimPx4v1_8/Sensor Model/Global reprojection ==
  x : Inport
  y : Inport  Port=2
  map_projection_reproject : MATLAB Function  TreatAsAtomicUnit=on
  lat : Outport
  lon : Outport  Port=2
  wires:
  y/1 -> map_projection_reproject/2(y)
  map_projection_reproject/2(lon) -> lon/1
  x/1 -> map_projection_reproject/1(x)
  map_projection_reproject/1(lat) -> lat/1

== system TestMultirotorSimPx4v1_8/Sensor Model/Gyroscope ==
  nuBody : Inport  Unit=rad/s
  Bias : Constant  Commented=on  Value=[0.0001;0.0001;0.0001]
  Delay1 : Delay  DelayLength=1  InitialConditionSource=Input port  SampleTime=1/400
      settings: InputPortMap=u0,p4
  Delay2 : Delay  DelayLength=1  InitialConditionSource=Input port  SampleTime=1/400
      settings: InputPortMap=u0,p4
  Delay4 : Delay  DelayLength=1  InitialConditionSource=Input port  SampleTime=1/400
      settings: InputPortMap=u0,p4
  Demux : Demux  Outputs=3
  Gain : Gain
  Mux : Mux  Inputs=3
  Sum2 : Sum  Inputs=++|
  gyro_rad : Outport  Unit=rad/s  SampleTime=1/400
  wires:
  Sum2/1 -> Demux/1
  Mux/1 -> gyro_rad/1
  Bias/1 -> Sum2/1
  nuBody/1 -> Gain/1
  Delay4/1 -> Mux/2
  Delay2/1 -> Mux/3
  Delay1/1 -> Mux/1
  Demux/1 -> Delay1/2, Delay1/1
  Demux/2 -> Delay4/2, Delay4/1
  Demux/3 -> Delay2/2, Delay2/1
  Gain/1 -> Sum2/2

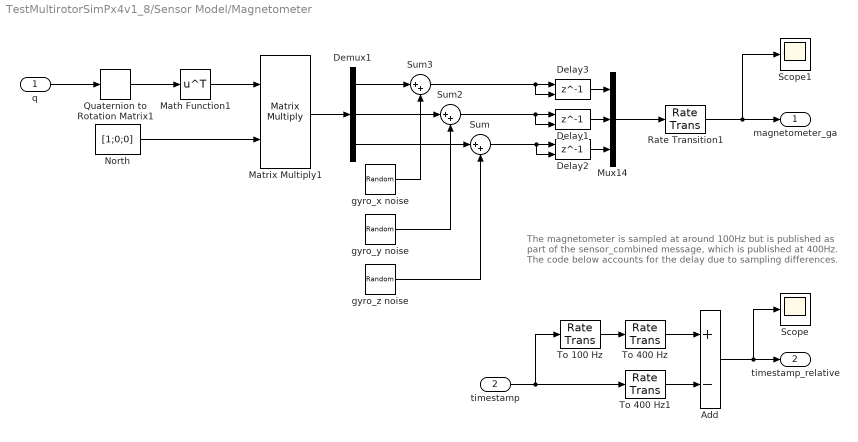
== system TestMultirotorSimPx4v1_8/Sensor Model/Magnetometer ==
  note: The magnetometer is sampled at around 100Hz but is published
      | as part of the sensor_combined message, which is published at
      | 400Hz. The code below accounts for the delay due to sampling
      | differences.
  q : Inport
  timestamp : Inport  Port=2
  Add : Sum  Inputs=+-
  Delay1 : Delay  DelayLength=1  InitialConditionSource=Input port  SampleTime=1/100
      settings: InputPortMap=u0,p4
  Delay2 : Delay  DelayLength=1  InitialConditionSource=Input port  SampleTime=1/100
      settings: InputPortMap=u0,p4
  Delay3 : Delay  DelayLength=1  InitialConditionSource=Input port  SampleTime=1/100
      settings: InputPortMap=u0,p4
  Demux1 : Demux  Outputs=3
  Math Function1 : Math  Operator=transpose  SaturateOnIntegerOverflow=on
  Matrix Multiply1 : Product  Multiplication=Matrix(*)
  Mux14 : Mux  Inputs=3
  North : Constant  Value=[1;0;0]
  Quaternion to Rotation Matrix1 : QuaternionLibrary/Quaternion to Rotation Matrix
  Rate Transition1 : RateTransition  Deterministic=off  OutPortSampleTime=1/100
  Scope : Scope
  Scope1 : Scope
  Sum : Sum  Inputs=|++
  Sum2 : Sum  Inputs=|++
  Sum3 : Sum  Inputs=|++
  To 100 Hz : RateTransition  OutPortSampleTime=1/100
  To 400 Hz : RateTransition  Deterministic=off  OutPortSampleTime=1/250
  To 400 Hz1 : RateTransition  OutPortSampleTime=1/400
  gyro_x noise : RandomNumber  Variance=0.001^2  SampleTime=1/400
  gyro_y noise : RandomNumber  Variance=0.001^2  SampleTime=1/400
  gyro_z noise : RandomNumber  Variance=0.001^2  SampleTime=1/400
  magnetometer_ga : Outport  Unit=G  SampleTime=1/250
  timestamp_relative : Outport  Port=2  Unit=µs  SampleTime=1/250
  wires:
  q/1 -> Quaternion to Rotation Matrix1/1
  Quaternion to Rotation Matrix1/1 -> Math Function1/1
  North/1 -> Matrix Multiply1/2
  Math Function1/1 -> Matrix Multiply1/1
  Add/1 -> timestamp_relative/1, Scope/1
  Matrix Multiply1/1 -> Demux1/1
  Demux1/1 -> Sum3/1
  Demux1/2 -> Sum2/1
  Demux1/3 -> Sum/1
  Sum/1 -> Delay2/2, Delay2/1
  gyro_z noise/1 -> Sum/2
  Sum2/1 -> Delay1/2, Delay1/1
  gyro_y noise/1 -> Sum2/2
  gyro_x noise/1 -> Sum3/2
  Mux14/1 -> Rate Transition1/1
  To 400 Hz1/1 -> Add/2
  To 100 Hz/1 -> To 400 Hz/1
  To 400 Hz/1 -> Add/1
  Rate Transition1/1 -> Scope1/1, magnetometer_ga/1
  timestamp/1 -> To 100 Hz/1, To 400 Hz1/1
  Delay3/1 -> Mux14/1
  Sum3/1 -> Delay3/2, Delay3/1
  Delay1/1 -> Mux14/2
  Delay2/1 -> Mux14/3

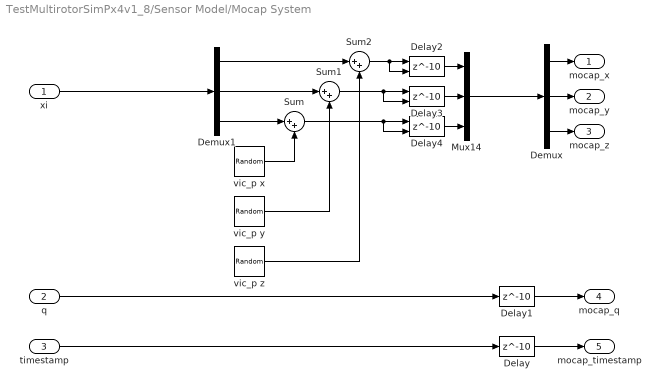
== system TestMultirotorSimPx4v1_8/Sensor Model/Mocap System ==
  xi : Inport
  q : Inport  Port=2
  timestamp : Inport  Port=3
  Delay : Delay  DelayLength=10  SampleTime=1/100
  Delay1 : Delay  DelayLength=10  SampleTime=1/100
  Delay2 : Delay  DelayLength=10  InitialConditionSource=Input port  SampleTime=1/100
      settings: InputPortMap=u0,p4
  Delay3 : Delay  DelayLength=10  InitialConditionSource=Input port  SampleTime=1/100
      settings: InputPortMap=u0,p4
  Delay4 : Delay  DelayLength=10  InitialConditionSource=Input port  SampleTime=1/100
      settings: InputPortMap=u0,p4
  Demux : Demux  Outputs=3
  Demux1 : Demux  Outputs=3
  Mux14 : Mux  Inputs=3
  Sum : Sum  Inputs=|++
  Sum1 : Sum  Inputs=|++
  Sum2 : Sum  Inputs=|++
  vic_p x : RandomNumber  Variance=0.001^2  SampleTime=0.01
  vic_p y : RandomNumber  Variance=0.001^2  SampleTime=0.01
  vic_p z : RandomNumber  Variance=0.001^2  SampleTime=0.01
  mocap_x : Outport
  mocap_y : Outport  Port=2
  mocap_z : Outport  Port=3
  mocap_q : Outport  Port=4
  mocap_timestamp : Outport  Port=5
  wires:
  q/1 -> Delay1/1
  timestamp/1 -> Delay/1
  Delay/1 -> mocap_timestamp/1
  Delay1/1 -> mocap_q/1
  Demux1/1 -> Sum2/1
  Demux1/2 -> Sum1/1
  xi/1 -> Demux1/1
  Demux1/3 -> Sum/1
  Sum/1 -> Delay4/2, Delay4/1
  vic_p x/1 -> Sum/2
  Sum1/1 -> Delay3/2, Delay3/1
  Sum2/1 -> Delay2/2, Delay2/1
  vic_p y/1 -> Sum1/2
  vic_p z/1 -> Sum2/2
  Demux/3 -> mocap_z/1
  Demux/2 -> mocap_y/1
  Demux/1 -> mocap_x/1
  Mux14/1 -> Demux/1
  Delay2/1 -> Mux14/1
  Delay3/1 -> Mux14/2
  Delay4/1 -> Mux14/3

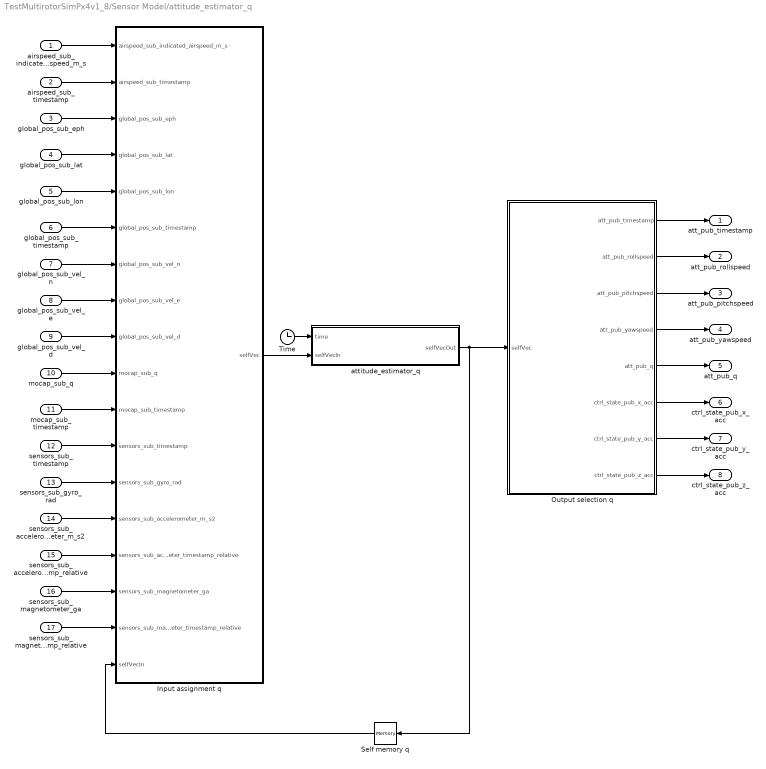
== system TestMultirotorSimPx4v1_8/Sensor Model/attitude_estimator_q ==
  airspeed_sub_indicated_airspeed_m_s : Inport
  airspeed_sub_timestamp : Inport  Port=2
  global_pos_sub_eph : Inport  Port=3
  global_pos_sub_lat : Inport  Port=4
  global_pos_sub_lon : Inport  Port=5
  global_pos_sub_timestamp : Inport  Port=6
  global_pos_sub_vel_n : Inport  Port=7
  global_pos_sub_vel_e : Inport  Port=8
  global_pos_sub_vel_d : Inport  Port=9
  mocap_sub_q : Inport  Port=10
  mocap_sub_timestamp : Inport  Port=11
  sensors_sub_timestamp : Inport  Port=12
  sensors_sub_gyro_rad : Inport  Port=13
  sensors_sub_accelerometer_m_s2 : Inport  Port=14
  sensors_sub_accelerometer_timestamp_relative : Inport  Port=15
  sensors_sub_magnetometer_ga : Inport  Port=16
  sensors_sub_magnetometer_timestamp_relative : Inport  Port=17
  Input assignment q : MATLAB Function  TreatAsAtomicUnit=on
  Output selection q : MATLAB Function  TreatAsAtomicUnit=on
  Self memory q : Memory  InitialCondition=[ATT_ACC_COMP, 0, 0, 0, 0, 0, 0, 0, FW_ARSP_MODE, 0, 0, 0, 0, 0, 0, 0, 0, INIT_Q(1), INIT_Q(2), INIT_Q(3), INIT_Q(4), ATT_BIAS_MAX, 0, 0, INIT_Q(1), INIT_Q(2), INIT_Q(3), INIT_Q(4), 0, 0, 0, 0, 0, 0, 0, 0, 0, 0, 0, 0, 0.02, 0, ATT_EXT_HDG_M, 0, 0, 0, 0, 0, 0, 0, 0, 0, 0, 0, 0, 0, 0, 0, 0, 0, 0, 0, 0, 0, 0, 0, 0, 0, 0, 0, 0, 0, 0, 0, 0, 0, 0, 0, 0, 0, 0, 0, 0, 0, 0, 0, 0, 0, 0, 0, 0, 0, 0, 0, 0, 0, 0, 0, 0, 0, 0, 0, 0, 0, 0, 0, 0, 0, 0, 0, 0, 0, 0, 0, 0, 0, 0, 0, 0, 0, 0, 0, 0, 0, 0, 0, 0, 0, 0, 0, 0, 0, ATT_MAG_DECL, ATT_MAG_DECL_A, 0, 0, 0, 0, 0, 0, 0, 0, 0, 0, 0, 0, 0, 0, 0, 0, 0, 0, 0, 0, 0, 0, INIT_Q(1), INIT_Q(2), INIT_Q(3), INIT_Q(4), 0, 0, 0, 0, 0, 0, 0, 0, 0, 0, 0, 0, 0, 0, 0, 0, 0, 0, 0, 0, 0, 0, 0, 0, 0, 0, 0, 0, 0, 0, 0, 0, 0, 0, 0, 0, 0, 0, 0, ATT_W_ACC, ATT_W_EXT_HDG, ATT_W_GYRO_BIAS, ATT_W_MAG, 0, 0]
  Time : Clock
  attitude_estimator_q : MATLAB Function  TreatAsAtomicUnit=on  SystemSampleTime=Q_SAMPLING_PERIOD
  att_pub_timestamp : Outport
  att_pub_rollspeed : Outport  Port=2
  att_pub_pitchspeed : Outport  Port=3
  att_pub_yawspeed : Outport  Port=4
  att_pub_q : Outport  Port=5
  ctrl_state_pub_x_acc : Outport  Port=6
  ctrl_state_pub_y_acc : Outport  Port=7
  ctrl_state_pub_z_acc : Outport  Port=8
  wires:
  Output selection q/8(ctrl_state_pub_z_acc) -> ctrl_state_pub_z_acc/1
  Output selection q/7(ctrl_state_pub_y_acc) -> ctrl_state_pub_y_acc/1
  Output selection q/6(ctrl_state_pub_x_acc) -> ctrl_state_pub_x_acc/1
  Output selection q/5(att_pub_q) -> att_pub_q/1
  Output selection q/4(att_pub_yawspeed) -> att_pub_yawspeed/1
  Output selection q/3(att_pub_pitchspeed) -> att_pub_pitchspeed/1
  Output selection q/2(att_pub_rollspeed) -> att_pub_rollspeed/1
  Output selection q/1(att_pub_timestamp) -> att_pub_timestamp/1
  sensors_sub_magnetometer_timestamp_relative/1 -> Input assignment q/17(sensors_sub_magnetometer_timestamp_relative)
  sensors_sub_magnetometer_ga/1 -> Input assignment q/16(sensors_sub_magnetometer_ga)
  sensors_sub_accelerometer_timestamp_relative/1 -> Input assignment q/15(sensors_sub_accelerometer_timestamp_relative)
  sensors_sub_accelerometer_m_s2/1 -> Input assignment q/14(sensors_sub_accelerometer_m_s2)
  sensors_sub_gyro_rad/1 -> Input assignment q/13(sensors_sub_gyro_rad)
  sensors_sub_timestamp/1 -> Input assignment q/12(sensors_sub_timestamp)
  mocap_sub_timestamp/1 -> Input assignment q/11(mocap_sub_timestamp)
  mocap_sub_q/1 -> Input assignment q/10(mocap_sub_q)
  global_pos_sub_vel_d/1 -> Input assignment q/9(global_pos_sub_vel_d)
  global_pos_sub_vel_e/1 -> Input assignment q/8(global_pos_sub_vel_e)
  global_pos_sub_vel_n/1 -> Input assignment q/7(global_pos_sub_vel_n)
  global_pos_sub_timestamp/1 -> Input assignment q/6(global_pos_sub_timestamp)
  global_pos_sub_lon/1 -> Input assignment q/5(global_pos_sub_lon)
  global_pos_sub_lat/1 -> Input assignment q/4(global_pos_sub_lat)
  global_pos_sub_eph/1 -> Input assignment q/3(global_pos_sub_eph)
  airspeed_sub_timestamp/1 -> Input assignment q/2(airspeed_sub_timestamp)
  airspeed_sub_indicated_airspeed_m_s/1 -> Input assignment q/1(airspeed_sub_indicated_airspeed_m_s)
  Time/1 -> attitude_estimator_q/1(time)
  Self memory q/1 -> Input assignment q/18(selfVecIn)
  attitude_estimator_q/1(selfVecOut) -> Self memory q/1, Output selection q/1(selfVec)
  Input assignment q/1(selfVec) -> attitude_estimator_q/2(selfVecIn)
